simulink model "ClosedLoopControl"  (R2023b)
settings: Solver=FixedStepDiscrete  StartTime=0.0  StopTime=inf  FixedStep=0.005  RelTol=1e-3
libraries: arduinolib x14, arduinosensorlib x4, eeGeneralControl x4, slpidlib x4, embeddedblockslib x2, simulink x2
settings Model: ExtModeTrigDuration=2  Creator=Jakob  LastModifiedBy=Jakob
settings OptimizationCC: EnhancedBackFolding=on  PassReuseOutputArgsAs=Individual arguments  ZeroExternalMemoryAtStartup=off  ZeroInternalMemoryAtStartup=off  MaxStackSize=64  OptimizeBlockOrder=speed  DifferentSizesBufferReuse=on  OptimizationCustomize=off  EfficientTunableParamExpr=on
settings DebuggingCC: ParameterTunabilityLossMsg=error
settings HardwareCC: ProdBitPerPointer=32  ProdBitPerSizeT=32  ProdBitPerPtrDiffT=32  ProdLargestAtomicInteger=Long  ProdLargestAtomicFloat=Double  ProdWordSize=32  ProdHWDeviceType=ARM Compatible->ARM Cortex
settings SFSimCC: MATLABDynamicMemAlloc=off
settings RTWCC: Description=Embedded Coder  SystemTargetFile=ert.tlc  HardwareBoard=ESP32-WROOM(Arduino Compatible)  TLCOptions="-aInlineSetEventsForThisBaseRateFcn=TLC_FALSE -aSuppressMultiTaskScheduler=TLC_FALSE  -aRateBasedStepFcn=0"  TemplateMakefile=ert_default_tmf  Toolchain=ESP32  BuildConfiguration=Faster Runs
settings CodeAppCC: ForceParamTrailComments=on  IgnoreCustomStorageClasses=off  OperatorAnnotations=on  SimulinkDataObjDesc=on  SFDataObjDesc=on  InsertBlockDesc=on
settings ERTTargetCC: SupportContinuousTime=on  SupportVariableSizeSignals=on  ExtModeTransport=3  ExtModeStaticAlloc=on  ExtModeAutomaticAllocSize=off  ExtModeStaticAllocSize=65536  ExtModeMexFile=ext_xcp  ExtModeIntrfLevel=Level2 - Open

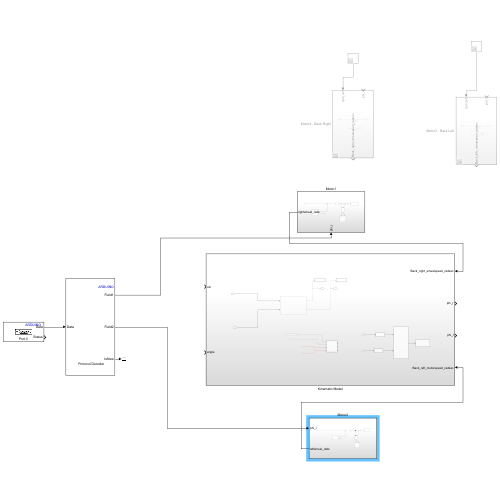
[thumbnail: Simulink's stored preview of the top-level diagram]
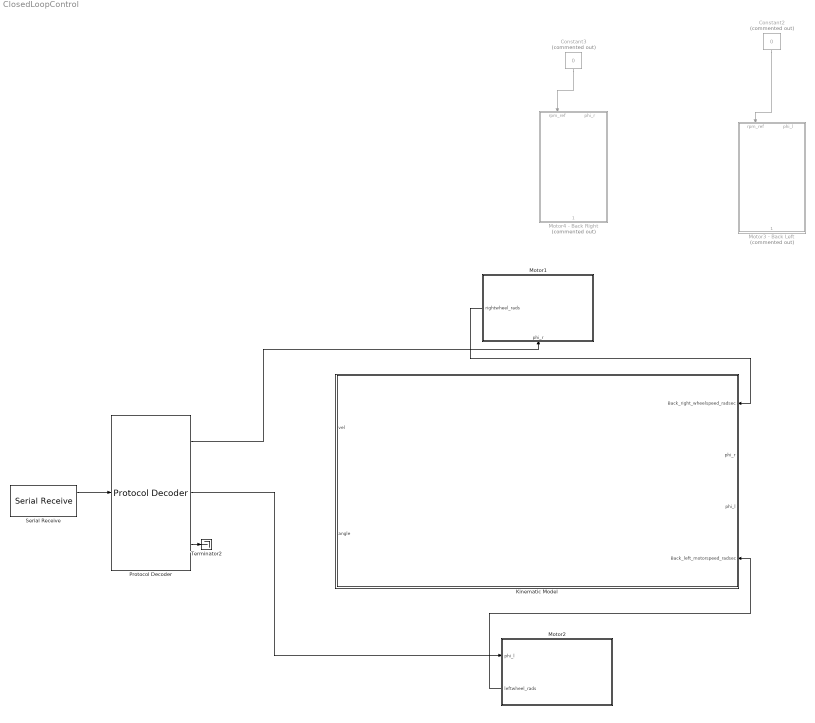
== system ClosedLoopControl ==
  Constant2 : Constant  Commented=on  Value=0
  Constant3 : Constant  Commented=on  Value=0
  Kinematic Model : Subsystem
      settings: PortSchema="{\"entries\":[{\"content\":{\"sides\":[{\"content\":{\"connectorIds\":[\"In1\",\"In2\"]},\"type\":\"ConnectorPlacement.EquallySpacedRectSide\",\"uuid\":\"bea487b3-b9a6-4df2-9051-f476a43b63d0\"},{\"content\":{\"connectorIds\":[\"In3\",\"Out1\",\"Out2\",\"In4\"],\"side\":\"RIGHT\"},\"type\":\"ConnectorPlacement.EquallySpacedRectSide\",\"uuid\":\"7b0ea2f1-f889-4d4a-8825-aa604977931d\"},{\"content\":{\"side\":\"TOP\"},\"type\":\"ConnectorPlacement.EquallySpacedRectSide\",\"uuid\":\"9098ab21-ef51-46af-af75-8fe6529eb13c\"}]},\"type\":\"ConnectorPlacement.EquallySpacedConnector\",\"uuid\":\"e0384f79-f267-486d-9835-e037e5e58d79\"}],\"packageUris\":[\"http://schema.mathworks.com/mf0/Connector/R2020b\"],\"version\":\"1.0\"}"
  Motor1 : Subsystem
      settings: PortSchema="{\"entries\":[{\"content\":{\"sides\":[{\"content\":{},\"type\":\"ConnectorPlacement.EquallySpacedRectSide\",\"uuid\":\"e90522e1-f096-4247-8870-f151728acb54\"},{\"content\":{\"connectorIds\":[\"Out1\"],\"side\":\"RIGHT\"},\"type\":\"ConnectorPlacement.EquallySpacedRectSide\",\"uuid\":\"14a2659e-e07a-4a14-8c7c-2c374d5141ee\"},{\"content\":{\"connectorIds\":[\"In1\"],\"side\":\"TOP\"},\"type\":\"ConnectorPlacement.EquallySpacedRectSide\",\"uuid\":\"95453d09-0c33-4ffa-a097-d1ecacc3e87c\"}]},\"type\":\"ConnectorPlacement.EquallySpacedConnector\",\"uuid\":\"f979addb-97c9-400b-8ed4-2cf1cffe9c36\"}],\"packageUris\":[\"http://schema.mathworks.com/mf0/Connector/R2020b\"],\"version\":\"1.0\"}"
  Motor2 : Subsystem
      settings: PortSchema="{\"entries\":[{\"content\":{\"sides\":[{\"content\":{},\"type\":\"ConnectorPlacement.EquallySpacedRectSide\",\"uuid\":\"e90522e1-f096-4247-8870-f151728acb54\"},{\"content\":{\"connectorIds\":[\"In1\",\"Out1\"],\"side\":\"RIGHT\"},\"type\":\"ConnectorPlacement.EquallySpacedRectSide\",\"uuid\":\"14a2659e-e07a-4a14-8c7c-2c374d5141ee\"},{\"content\":{\"side\":\"TOP\"},\"type\":\"ConnectorPlacement.EquallySpacedRectSide\",\"uuid\":\"95453d09-0c33-4ffa-a097-d1ecacc3e87c\"}]},\"type\":\"ConnectorPlacement.EquallySpacedConnector\",\"uuid\":\"f979addb-97c9-400b-8ed4-2cf1cffe9c36\"}],\"packageUris\":[\"http://schema.mathworks.com/mf0/Connector/R2020b\"],\"version\":\"1.0\"}"
  Motor3 - Back Left : Subsystem  Commented=on
  Motor4 - Back Right : Subsystem  Commented=on
  Protocol Decoder : embeddedblockslib/Protocol Decoder  IsParseCSV=off  Header=['$']  FieldTable={ 'Field1', '1', 'single', 'Little endian'; 'Field2', '1', 'single', 'Little endian' }  IsVariableSizeLastField=off  MaxVariableSizeFieldLength=[]  IsChecksumRequired=off  ChecksumAlgorithm=XOR of bytes  ChecksumSize=[]  TerminatorOption=<none>  CustomTerminatorVal=[]  IsInputLengthAvailable=off  Logo=ARDUINO
      settings: LibrarySourceBlock=arduinolib/Protocol Decoder
  Serial Receive : arduinolib/Serial Receive  isARMArch=off  portNumber=0  DataType=uint8  Datalength=9  SampleTime=0.005  showOutStatus=on  blockPlatform=arduino
  Terminator2 : Terminator
  wires:
  Constant2/1 -> Motor3 - Back Left/1(rpm_ref)
  Constant3/1 -> Motor4 - Back Right/1(rpm_ref)
  Motor2/1(leftwheel_rads) -> Kinematic Model/4(Back_left_motorspeed_radsec)
  Motor1/1(rightwheel_rads) -> Kinematic Model/3(Back_right_wheelspeed_radsec)
  Protocol Decoder/3 -> Terminator2/1
  Serial Receive/1 -> Protocol Decoder/1
  Protocol Decoder/1 -> Motor1/1(phi_r)
  Protocol Decoder/2 -> Motor2/1(phi_l)

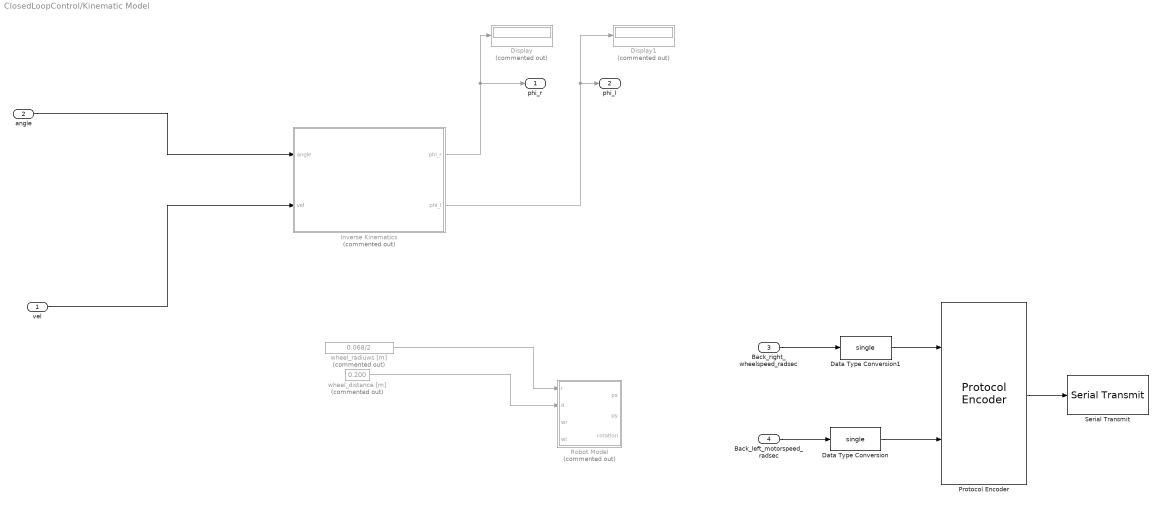
== system ClosedLoopControl/Kinematic Model ==
  vel : Inport
  angle : Inport  Port=2
  Back_right_wheelspeed_radsec : Inport  Port=3
  Back_left_motorspeed_radsec : Inport  Port=4
  Data Type Conversion : DataTypeConversion  OutDataTypeStr=single  SaturateOnIntegerOverflow=off  RndMeth=Floor
  Data Type Conversion1 : DataTypeConversion  OutDataTypeStr=single  SaturateOnIntegerOverflow=off  RndMeth=Floor
  Display : Display  Commented=on
  Display1 : Display  Commented=on
  Inverse Kinematics : Subsystem  Commented=on
  Protocol Encoder : embeddedblockslib/Protocol Encoder  Header=['$']  FieldTable={ 'Field1', '1', 'single', 'Little endian'; 'Field2', '1', 'single', 'Little endian' }  IsChecksumRequired=off  ChecksumAlgorithm=XOR of bytes  ChecksumSize=[]  TerminatorOption=<none>  CustomTerminatorVal=[]  Logo=ARDUINO
      settings: LibrarySourceBlock=arduinolib/Protocol Encoder
  Robot Model : Subsystem  Commented=on
  Serial Transmit : arduinolib/Serial Transmit  portNumber=0  sendmode=write  sendformat=Decimal  floatprecision=2  blockPlatform=arduino
  wheel_distance [m] : Constant  Commented=on  Value=0.200
  wheel_radiuws [m] : Constant  Commented=on  Value=0.068/2
  phi_r : Outport
  phi_l : Outport  Port=2
  wires:
  wheel_radiuws [m]/1 -> Robot Model/1(r)
  wheel_distance [m]/1 -> Robot Model/2(d)
  Inverse Kinematics/1(phi_r) -> Display/1, phi_r/1
  Inverse Kinematics/2(phi_l) -> Display1/1, phi_l/1
  ? -> Robot Model/3(wr)
  ? -> Robot Model/4(wl)
  vel/1 -> Inverse Kinematics/2(vel)
  angle/1 -> Inverse Kinematics/1(angle)
  Protocol Encoder/1 -> Serial Transmit/1
  Data Type Conversion/1 -> Protocol Encoder/2
  Data Type Conversion1/1 -> Protocol Encoder/1
  Back_right_wheelspeed_radsec/1 -> Data Type Conversion1/1
  Back_left_motorspeed_radsec/1 -> Data Type Conversion/1

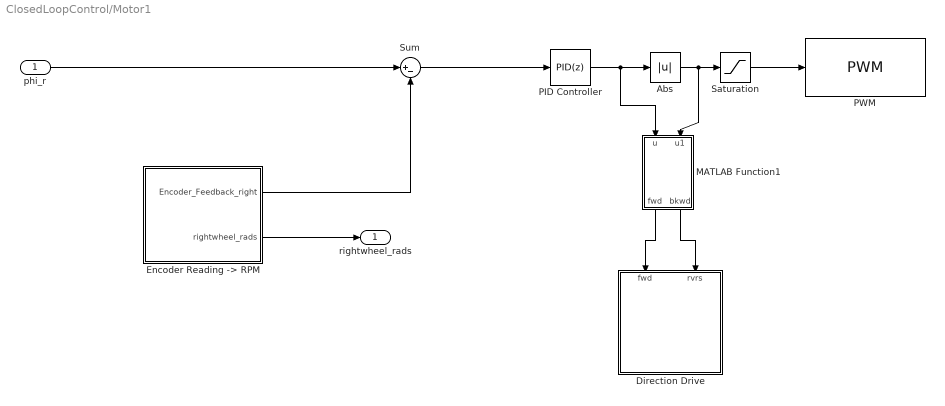
== system ClosedLoopControl/Motor1 ==
  phi_r : Inport
  Abs : Abs  SaturateOnIntegerOverflow=off
  Direction Drive : Subsystem
  "Encoder Reading -> RPM" : Subsystem
  MATLAB Function1 : MATLAB Function  TreatAsAtomicUnit=on
  PID Controller : slpidlib/PID Controller  Controller=PID  Form=Parallel  TimeDomain=Discrete-time  UseExternalTs=off  SampleTime=-1  IntegratorMethod=Forward Euler  FilterMethod=Forward Euler  ControllerParametersSource=internal  P=25  I=350  UseKiTs=off  D=0  N=100  UseFilter=on  TunerSelectOption=Transfer Function Based (PID Tuner App)  InitialConditionSource=internal  InitialConditionForIntegrator=0  InitialConditionForFilter=0  DifferentiatorICPrevScaledInput=0  ExternalReset=none  TrackingMode=off  Kt=1  LimitOutput=off  SatLimitsSource=internal  UpperSaturationLimit=inf  LowerSaturationLimit=-inf  LinearizeAsGain=on  AntiWindupMode=none  Kb=1  LimitIntegrator=off  UpperIntegratorSaturationLimit=inf  LowerIntegratorSaturationLimit=-inf  POutMin=[]  POutMax=[]  IOutMin=[]  IOutMax=[]  DOutMin=[]  DOutMax=[]  NOutMin=[]  NOutMax=[]  SumOutMin=[]  SumOutMax=[]  SaturationOutMin=[]  SaturationOutMax=[]  PParamMin=[]  PParamMax=[]  IParamMin=[]  IParamMax=[]  DParamMin=[]  DParamMax=[]  NParamMin=[]  NParamMax=[]  KbParamMin=[]  KbParamMax=[]  KtParamMin=[]  KtParamMax=[]  KbOutMin=[]  KbOutMax=[]  KtOutMin=[]  KtOutMax=[]  IntegratorOutMin=[]  IntegratorOutMax=[]  FilterOutMin=[]  FilterOutMax=[]  SumI1OutMin=[]  SumI1OutMax=[]  SumI2OutMin=[]  SumI2OutMax=[]  SumI3OutMin=[]  SumI3OutMax=[]  SumI4OutMin=[]  SumI4OutMax=[]  SumDOutMin=[]  SumDOutMax=[]  DifferentiatorOutMin=[]  DifferentiatorOutMax=[]  FilterDiffOutCoefMin=[]  FilterDiffOutCoefMax=[]  ReciprocalOutMin=[]  ReciprocalOutMax=[]  SumDenOutMin=[]  SumDenOutMax=[]  SumNumOutMin=[]  SumNumOutMax=[]  DivideOutMin=[]  DivideOutMax=[]  UdiffTsProdOutMin=[]  UdiffTsProdOutMax=[]  NTsProdOutMin=[]  NTsProdOutMax=[]  UintegralTsProdOutMin=[]  UintegralTsProdOutMax=[]  UngainTsProdOutMin=[]  UngainTsProdOutMax=[]  ClampingZeroOutDataTypeStr=Inherit: Inherit via back propagation  ClampingZeroOutMin=[]  ClampingZeroOutMax=[]  FilterDenConstantOutDataTypeStr=Inherit: Inherit via back propagation  FilterDenConstantOutMin=[]  FilterDenConstantOutMax=[]  PCopyOutDataTypeStr=Inherit: Inherit via back propagation  PCopyOutMin=[]  PCopyOutMax=[]  NCopyOutDataTypeStr=Inherit: Inherit via back propagation  NCopyOutMin=[]  NCopyOutMax=[]  IntegratorContinuousStateAttributes=''  IntegratorStateMustResolveToSignalObject=off  IntegratorRTWStateStorageClass=Auto  FilterContinuousStateAttributes=''  FilterStateMustResolveToSignalObject=off  FilterRTWStateStorageClass=Auto  ParallelPVariant=InternalParameters  IdealPVariant=Disabled  IVariant=InternalParameters  DVariant=InternalParameters  IntegratorVariant=Discrete  SatVariant=Disabled  AWVariant=Passthrough  PCopyVariant=Disabled  TRVariant=Disabled  FdbkBlocksVariant=Forward  IdealPFdbkVariant=Disabled  SatFdbkVariant=Disabled  DerivativeFilterVariant=ForwardEulerFilter  NVariant=InternalParameters  NCopyVariant=Disabled  FilterICVariant=InternalICsFilter  IntegratorICVariant=InternalICs  ExternalResetVariant=Disabled  TRSumVariant=Passthrough  SumFdbkVariant=Disabled  SumVariant=Sum_PID  TsampFilterVariant=InternalTs  TsampNgainVariant=Passthrough  TsampIntegralVariant=Disabled_SignalSpec  ExternalSaturationOutDataTypeStr=Inherit: Same as second input
  PWM : arduinolib/PWM  pinNumber=18  frequencyType=Default  desiredFrequency=490.2  achievableFrequency=490.2
  Saturation : Saturate  UpperLimit=255  LowerLimit=0
  Sum : Sum  Inputs=|+-
  rightwheel_rads : Outport
  wires:
  PID Controller/1 -> MATLAB Function1/1(u), Abs/1
  Sum/1 -> PID Controller/1
  Saturation/1 -> PWM/1
  "Encoder Reading -> RPM"/2(rightwheel_rads) -> rightwheel_rads/1
  phi_r/1 -> Sum/1
  "Encoder Reading -> RPM"/1(Encoder_Feedback_right) -> Sum/2
  Abs/1 -> MATLAB Function1/2(u1), Saturation/1
  MATLAB Function1/1(fwd) -> Direction Drive/1(fwd)
  MATLAB Function1/2(bkwd) -> Direction Drive/2(rvrs)

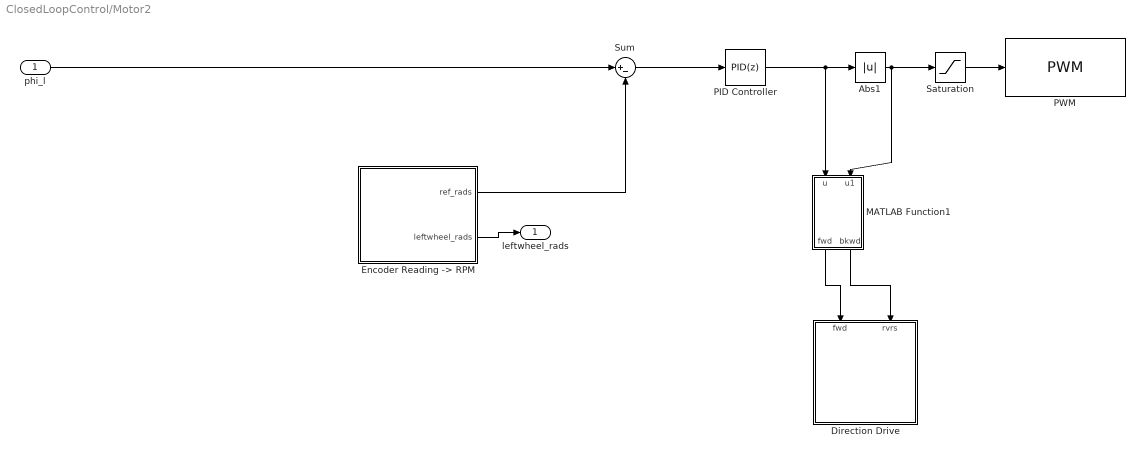
== system ClosedLoopControl/Motor2 ==
  phi_l : Inport
  Abs1 : Abs  SaturateOnIntegerOverflow=off
  Direction Drive : Subsystem
  "Encoder Reading -> RPM" : Subsystem
  MATLAB Function1 : MATLAB Function  TreatAsAtomicUnit=on
  PID Controller : slpidlib/PID Controller  Controller=PID  Form=Parallel  TimeDomain=Discrete-time  UseExternalTs=off  SampleTime=-1  IntegratorMethod=Forward Euler  FilterMethod=Forward Euler  ControllerParametersSource=internal  P=25  I=350  UseKiTs=off  D=0  N=100  UseFilter=on  TunerSelectOption=Transfer Function Based (PID Tuner App)  InitialConditionSource=internal  InitialConditionForIntegrator=0  InitialConditionForFilter=0  DifferentiatorICPrevScaledInput=0  ExternalReset=none  TrackingMode=off  Kt=1  LimitOutput=off  SatLimitsSource=internal  UpperSaturationLimit=inf  LowerSaturationLimit=-inf  LinearizeAsGain=on  AntiWindupMode=none  Kb=1  LimitIntegrator=off  UpperIntegratorSaturationLimit=inf  LowerIntegratorSaturationLimit=-inf  POutMin=[]  POutMax=[]  IOutMin=[]  IOutMax=[]  DOutMin=[]  DOutMax=[]  NOutMin=[]  NOutMax=[]  SumOutMin=[]  SumOutMax=[]  SaturationOutMin=[]  SaturationOutMax=[]  PParamMin=[]  PParamMax=[]  IParamMin=[]  IParamMax=[]  DParamMin=[]  DParamMax=[]  NParamMin=[]  NParamMax=[]  KbParamMin=[]  KbParamMax=[]  KtParamMin=[]  KtParamMax=[]  KbOutMin=[]  KbOutMax=[]  KtOutMin=[]  KtOutMax=[]  IntegratorOutMin=[]  IntegratorOutMax=[]  FilterOutMin=[]  FilterOutMax=[]  SumI1OutMin=[]  SumI1OutMax=[]  SumI2OutMin=[]  SumI2OutMax=[]  SumI3OutMin=[]  SumI3OutMax=[]  SumI4OutMin=[]  SumI4OutMax=[]  SumDOutMin=[]  SumDOutMax=[]  DifferentiatorOutMin=[]  DifferentiatorOutMax=[]  FilterDiffOutCoefMin=[]  FilterDiffOutCoefMax=[]  ReciprocalOutMin=[]  ReciprocalOutMax=[]  SumDenOutMin=[]  SumDenOutMax=[]  SumNumOutMin=[]  SumNumOutMax=[]  DivideOutMin=[]  DivideOutMax=[]  UdiffTsProdOutMin=[]  UdiffTsProdOutMax=[]  NTsProdOutMin=[]  NTsProdOutMax=[]  UintegralTsProdOutMin=[]  UintegralTsProdOutMax=[]  UngainTsProdOutMin=[]  UngainTsProdOutMax=[]  ClampingZeroOutDataTypeStr=Inherit: Inherit via back propagation  ClampingZeroOutMin=[]  ClampingZeroOutMax=[]  FilterDenConstantOutDataTypeStr=Inherit: Inherit via back propagation  FilterDenConstantOutMin=[]  FilterDenConstantOutMax=[]  PCopyOutDataTypeStr=Inherit: Inherit via back propagation  PCopyOutMin=[]  PCopyOutMax=[]  NCopyOutDataTypeStr=Inherit: Inherit via back propagation  NCopyOutMin=[]  NCopyOutMax=[]  IntegratorContinuousStateAttributes=''  IntegratorStateMustResolveToSignalObject=off  IntegratorRTWStateStorageClass=Auto  FilterContinuousStateAttributes=''  FilterStateMustResolveToSignalObject=off  FilterRTWStateStorageClass=Auto  ParallelPVariant=InternalParameters  IdealPVariant=Disabled  IVariant=InternalParameters  DVariant=InternalParameters  IntegratorVariant=Discrete  SatVariant=Disabled  AWVariant=Passthrough  PCopyVariant=Disabled  TRVariant=Disabled  FdbkBlocksVariant=Forward  IdealPFdbkVariant=Disabled  SatFdbkVariant=Disabled  DerivativeFilterVariant=ForwardEulerFilter  NVariant=InternalParameters  NCopyVariant=Disabled  FilterICVariant=InternalICsFilter  IntegratorICVariant=InternalICs  ExternalResetVariant=Disabled  TRSumVariant=Passthrough  SumFdbkVariant=Disabled  SumVariant=Sum_PID  TsampFilterVariant=InternalTs  TsampNgainVariant=Passthrough  TsampIntegralVariant=Disabled_SignalSpec  ExternalSaturationOutDataTypeStr=Inherit: Same as second input
  PWM : arduinolib/PWM  pinNumber=15  frequencyType=Default  desiredFrequency=490.2  achievableFrequency=490.2
  Saturation : Saturate  UpperLimit=255  LowerLimit=0
  Sum : Sum  Inputs=|+-
  leftwheel_rads : Outport
  wires:
  PID Controller/1 -> MATLAB Function1/1(u), Abs1/1
  Sum/1 -> PID Controller/1
  Saturation/1 -> PWM/1
  "Encoder Reading -> RPM"/2(leftwheel_rads) -> leftwheel_rads/1
  phi_l/1 -> Sum/1
  "Encoder Reading -> RPM"/1(ref_rads) -> Sum/2
  Abs1/1 -> MATLAB Function1/2(u1), Saturation/1
  MATLAB Function1/1(fwd) -> Direction Drive/1(fwd)
  MATLAB Function1/2(bkwd) -> Direction Drive/2(rvrs)

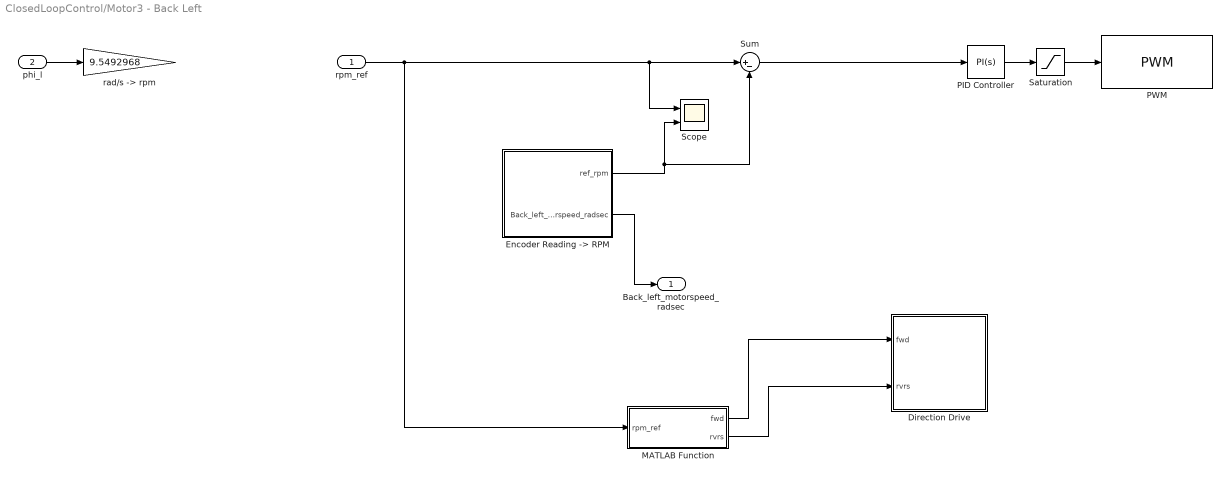
== system ClosedLoopControl/Motor3 - Back Left ==
  rpm_ref : Inport
  phi_l : Inport  Port=2
  Direction Drive : Subsystem
  "Encoder Reading -> RPM" : Subsystem
  MATLAB Function : MATLAB Function  TreatAsAtomicUnit=on
  PID Controller : slpidlib/PID Controller  Controller=PI  Form=Ideal  TimeDomain=Continuous-time  UseExternalTs=off  SampleTime=-1  IntegratorMethod=Forward Euler  FilterMethod=Forward Euler  ControllerParametersSource=internal  P=85  I=0.5  UseKiTs=off  D=0  N=100  UseFilter=on  TunerSelectOption=Transfer Function Based (PID Tuner App)  InitialConditionSource=internal  InitialConditionForIntegrator=0  InitialConditionForFilter=0  DifferentiatorICPrevScaledInput=0  ExternalReset=none  TrackingMode=off  Kt=1  LimitOutput=off  SatLimitsSource=internal  UpperSaturationLimit=inf  LowerSaturationLimit=-inf  LinearizeAsGain=on  AntiWindupMode=none  Kb=1  LimitIntegrator=off  UpperIntegratorSaturationLimit=inf  LowerIntegratorSaturationLimit=-inf  POutMin=[]  POutMax=[]  IOutMin=[]  IOutMax=[]  DOutMin=[]  DOutMax=[]  NOutMin=[]  NOutMax=[]  SumOutMin=[]  SumOutMax=[]  SaturationOutMin=[]  SaturationOutMax=[]  PParamMin=[]  PParamMax=[]  IParamMin=[]  IParamMax=[]  DParamMin=[]  DParamMax=[]  NParamMin=[]  NParamMax=[]  KbParamMin=[]  KbParamMax=[]  KtParamMin=[]  KtParamMax=[]  KbOutMin=[]  KbOutMax=[]  KtOutMin=[]  KtOutMax=[]  IntegratorOutMin=[]  IntegratorOutMax=[]  FilterOutMin=[]  FilterOutMax=[]  SumI1OutMin=[]  SumI1OutMax=[]  SumI2OutMin=[]  SumI2OutMax=[]  SumI3OutMin=[]  SumI3OutMax=[]  SumI4OutMin=[]  SumI4OutMax=[]  SumDOutMin=[]  SumDOutMax=[]  DifferentiatorOutMin=[]  DifferentiatorOutMax=[]  FilterDiffOutCoefMin=[]  FilterDiffOutCoefMax=[]  ReciprocalOutMin=[]  ReciprocalOutMax=[]  SumDenOutMin=[]  SumDenOutMax=[]  SumNumOutMin=[]  SumNumOutMax=[]  DivideOutMin=[]  DivideOutMax=[]  UdiffTsProdOutMin=[]  UdiffTsProdOutMax=[]  NTsProdOutMin=[]  NTsProdOutMax=[]  UintegralTsProdOutMin=[]  UintegralTsProdOutMax=[]  UngainTsProdOutMin=[]  UngainTsProdOutMax=[]  ClampingZeroOutDataTypeStr=Inherit: Inherit via back propagation  ClampingZeroOutMin=[]  ClampingZeroOutMax=[]  FilterDenConstantOutDataTypeStr=Inherit: Inherit via back propagation  FilterDenConstantOutMin=[]  FilterDenConstantOutMax=[]  PCopyOutDataTypeStr=Inherit: Inherit via back propagation  PCopyOutMin=[]  PCopyOutMax=[]  NCopyOutDataTypeStr=Inherit: Inherit via back propagation  NCopyOutMin=[]  NCopyOutMax=[]  IntegratorContinuousStateAttributes=''  IntegratorStateMustResolveToSignalObject=off  IntegratorRTWStateStorageClass=Auto  FilterContinuousStateAttributes=''  FilterStateMustResolveToSignalObject=off  FilterRTWStateStorageClass=Auto  ParallelPVariant=Passthrough  IdealPVariant=InternalParameters  IVariant=InternalParameters  DVariant=Disabled  IntegratorVariant=Continuous  SatVariant=Disabled  AWVariant=Passthrough  PCopyVariant=Disabled  TRVariant=Disabled  FdbkBlocksVariant=Forward  IdealPFdbkVariant=Disabled  SatFdbkVariant=Disabled  DerivativeFilterVariant=Disabled  NVariant=Disabled  NCopyVariant=Disabled_SignalSpec  FilterICVariant=Disabled  IntegratorICVariant=InternalICs  ExternalResetVariant=Disabled  TRSumVariant=Passthrough  SumFdbkVariant=Disabled  SumVariant=Sum_PI  TsampFilterVariant=InternalTs  TsampNgainVariant=Passthrough  TsampIntegralVariant=Disabled_SignalSpec  ExternalSaturationOutDataTypeStr=Inherit: Same as second input
  PWM : arduinolib/PWM  pinNumber=32  frequencyType=Default  desiredFrequency=490.2  achievableFrequency=490.2
  Saturation : Saturate  UpperLimit=255  LowerLimit=-255
  Scope : Scope  NumInputPorts=2
  Sum : Sum  Inputs=|+-
  "rad/s -> rpm" : Gain  Gain=9.5492968
  Back_left_motorspeed_radsec : Outport
  wires:
  PID Controller/1 -> Saturation/1
  Sum/1 -> PID Controller/1
  "Encoder Reading -> RPM"/1(ref_rpm) -> Sum/2, Scope/2
  phi_l/1 -> "rad/s -> rpm"/1
  Saturation/1 -> PWM/1
  "Encoder Reading -> RPM"/2(Back_left_motorspeed_radsec) -> Back_left_motorspeed_radsec/1
  MATLAB Function/1(fwd) -> Direction Drive/1(fwd)
  MATLAB Function/2(rvrs) -> Direction Drive/2(rvrs)
  rpm_ref/1 -> MATLAB Function/1(rpm_ref), Scope/1, Sum/1

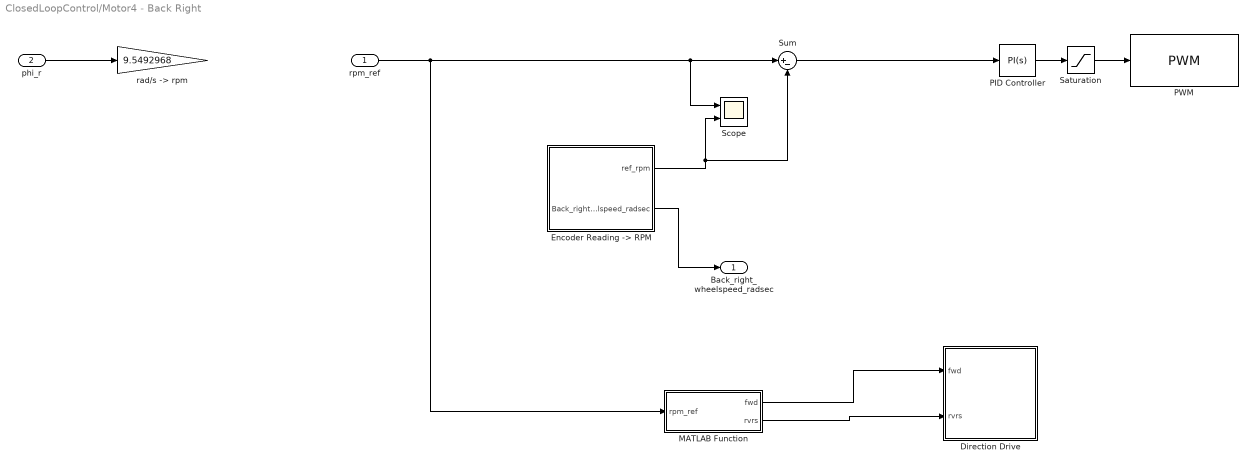
== system ClosedLoopControl/Motor4 - Back Right ==
  rpm_ref : Inport
  phi_r : Inport  Port=2
  Direction Drive : Subsystem
  "Encoder Reading -> RPM" : Subsystem
  MATLAB Function : MATLAB Function  TreatAsAtomicUnit=on
  PID Controller : slpidlib/PID Controller  Controller=PI  Form=Ideal  TimeDomain=Continuous-time  UseExternalTs=off  SampleTime=-1  IntegratorMethod=Forward Euler  FilterMethod=Forward Euler  ControllerParametersSource=internal  P=85  I=0.5  UseKiTs=off  D=0  N=100  UseFilter=on  TunerSelectOption=Transfer Function Based (PID Tuner App)  InitialConditionSource=internal  InitialConditionForIntegrator=0  InitialConditionForFilter=0  DifferentiatorICPrevScaledInput=0  ExternalReset=none  TrackingMode=off  Kt=1  LimitOutput=off  SatLimitsSource=internal  UpperSaturationLimit=inf  LowerSaturationLimit=-inf  LinearizeAsGain=on  AntiWindupMode=none  Kb=1  LimitIntegrator=off  UpperIntegratorSaturationLimit=inf  LowerIntegratorSaturationLimit=-inf  POutMin=[]  POutMax=[]  IOutMin=[]  IOutMax=[]  DOutMin=[]  DOutMax=[]  NOutMin=[]  NOutMax=[]  SumOutMin=[]  SumOutMax=[]  SaturationOutMin=[]  SaturationOutMax=[]  PParamMin=[]  PParamMax=[]  IParamMin=[]  IParamMax=[]  DParamMin=[]  DParamMax=[]  NParamMin=[]  NParamMax=[]  KbParamMin=[]  KbParamMax=[]  KtParamMin=[]  KtParamMax=[]  KbOutMin=[]  KbOutMax=[]  KtOutMin=[]  KtOutMax=[]  IntegratorOutMin=[]  IntegratorOutMax=[]  FilterOutMin=[]  FilterOutMax=[]  SumI1OutMin=[]  SumI1OutMax=[]  SumI2OutMin=[]  SumI2OutMax=[]  SumI3OutMin=[]  SumI3OutMax=[]  SumI4OutMin=[]  SumI4OutMax=[]  SumDOutMin=[]  SumDOutMax=[]  DifferentiatorOutMin=[]  DifferentiatorOutMax=[]  FilterDiffOutCoefMin=[]  FilterDiffOutCoefMax=[]  ReciprocalOutMin=[]  ReciprocalOutMax=[]  SumDenOutMin=[]  SumDenOutMax=[]  SumNumOutMin=[]  SumNumOutMax=[]  DivideOutMin=[]  DivideOutMax=[]  UdiffTsProdOutMin=[]  UdiffTsProdOutMax=[]  NTsProdOutMin=[]  NTsProdOutMax=[]  UintegralTsProdOutMin=[]  UintegralTsProdOutMax=[]  UngainTsProdOutMin=[]  UngainTsProdOutMax=[]  ClampingZeroOutDataTypeStr=Inherit: Inherit via back propagation  ClampingZeroOutMin=[]  ClampingZeroOutMax=[]  FilterDenConstantOutDataTypeStr=Inherit: Inherit via back propagation  FilterDenConstantOutMin=[]  FilterDenConstantOutMax=[]  PCopyOutDataTypeStr=Inherit: Inherit via back propagation  PCopyOutMin=[]  PCopyOutMax=[]  NCopyOutDataTypeStr=Inherit: Inherit via back propagation  NCopyOutMin=[]  NCopyOutMax=[]  IntegratorContinuousStateAttributes=''  IntegratorStateMustResolveToSignalObject=off  IntegratorRTWStateStorageClass=Auto  FilterContinuousStateAttributes=''  FilterStateMustResolveToSignalObject=off  FilterRTWStateStorageClass=Auto  ParallelPVariant=Passthrough  IdealPVariant=InternalParameters  IVariant=InternalParameters  DVariant=Disabled  IntegratorVariant=Continuous  SatVariant=Disabled  AWVariant=Passthrough  PCopyVariant=Disabled  TRVariant=Disabled  FdbkBlocksVariant=Forward  IdealPFdbkVariant=Disabled  SatFdbkVariant=Disabled  DerivativeFilterVariant=Disabled  NVariant=Disabled  NCopyVariant=Disabled_SignalSpec  FilterICVariant=Disabled  IntegratorICVariant=InternalICs  ExternalResetVariant=Disabled  TRSumVariant=Passthrough  SumFdbkVariant=Disabled  SumVariant=Sum_PI  TsampFilterVariant=InternalTs  TsampNgainVariant=Passthrough  TsampIntegralVariant=Disabled_SignalSpec  ExternalSaturationOutDataTypeStr=Inherit: Same as second input
  PWM : arduinolib/PWM  pinNumber=13  frequencyType=Default  desiredFrequency=490.2  achievableFrequency=490.2
  Saturation : Saturate  UpperLimit=255  LowerLimit=-255
  Scope : Scope  NumInputPorts=2
  Sum : Sum  Inputs=|+-
  "rad/s -> rpm" : Gain  Gain=9.5492968
  Back_right_wheelspeed_radsec : Outport
  wires:
  PID Controller/1 -> Saturation/1
  Sum/1 -> PID Controller/1
  "Encoder Reading -> RPM"/1(ref_rpm) -> Sum/2, Scope/2
  phi_r/1 -> "rad/s -> rpm"/1
  Saturation/1 -> PWM/1
  "Encoder Reading -> RPM"/2(Back_right_wheelspeed_radsec) -> Back_right_wheelspeed_radsec/1
  MATLAB Function/1(fwd) -> Direction Drive/1(fwd)
  MATLAB Function/2(rvrs) -> Direction Drive/2(rvrs)
  rpm_ref/1 -> MATLAB Function/1(rpm_ref), Scope/1, Sum/1

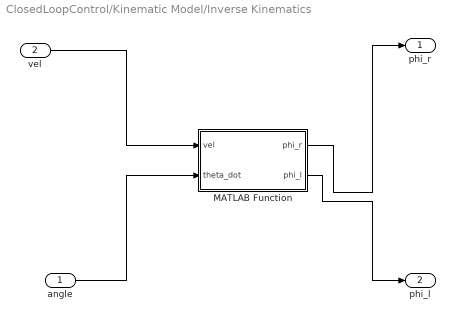
== system ClosedLoopControl/Kinematic Model/Inverse Kinematics ==
  angle : Inport
  vel : Inport  Port=2
  MATLAB Function : MATLAB Function  TreatAsAtomicUnit=on
  phi_r : Outport
  phi_l : Outport  Port=2
  wires:
  angle/1 -> MATLAB Function/2(theta_dot)
  vel/1 -> MATLAB Function/1(vel)
  MATLAB Function/1(phi_r) -> phi_r/1
  MATLAB Function/2(phi_l) -> phi_l/1

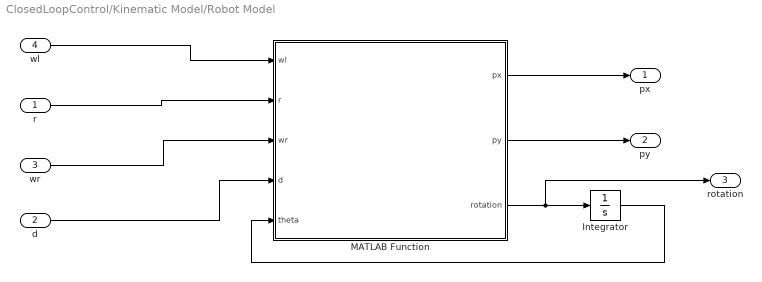
== system ClosedLoopControl/Kinematic Model/Robot Model ==
  r : Inport
  d : Inport  Port=2
  wr : Inport  Port=3
  wl : Inport  Port=4
  Integrator : Integrator
  MATLAB Function : MATLAB Function  TreatAsAtomicUnit=on
  px : Outport
  py : Outport  Port=2
  rotation : Outport  Port=3
  wires:
  wl/1 -> MATLAB Function/1(wl)
  r/1 -> MATLAB Function/2(r)
  d/1 -> MATLAB Function/4(d)
  wr/1 -> MATLAB Function/3(wr)
  MATLAB Function/1(px) -> px/1
  MATLAB Function/2(py) -> py/1
  MATLAB Function/3(rotation) -> rotation/1, Integrator/1
  Integrator/1 -> MATLAB Function/5(theta)

== system ClosedLoopControl/Motor1/Direction Drive ==
  fwd : Inport
  rvrs : Inport  Port=2
  Forward : arduinolib/Digital Output  pinNumber=5  Direction=output  blockPlatform=arduino
  Reverse : arduinolib/Digital Output  pinNumber=17  Direction=output  blockPlatform=arduino
  wires:
  rvrs/1 -> Reverse/1
  fwd/1 -> Forward/1

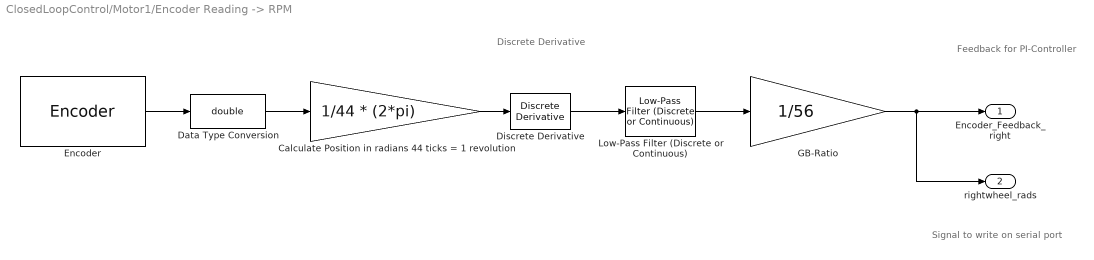
== system ClosedLoopControl/Motor1/Encoder Reading -> RPM ==
  note: Signal to write on serial port
  note: Feedback for PI-Controller
  note: Discrete Derivative
  Calculate Position in radians 44 ticks = 1 revolution : Gain  Gain=1/44 * (2*pi)
  Data Type Conversion : DataTypeConversion  OutDataTypeStr=double  SaturateOnIntegerOverflow=off  RndMeth=Floor
  Discrete Derivative : simulink/Discrete/Discrete Derivative  gainval=1.0  ICPrevScaledInput=0.0  OutMin=[]  OutMax=[]  OutDataType=fixdt(1, 16)  OutScaling=2^-10  DoSatur=off
  Encoder : arduinosensorlib/Encoder  InputA=19  InputB=23  Mode=No reset  SampleTime=-1
  GB-Ratio : Gain  Gain=1/56
  Low-Pass Filter (Discrete or Continuous) : eeGeneralControl/Low-Pass Filter (Discrete or Continuous)  K=1  T=0.05  B=inf  A=-inf  init_option=Inherited from block input  x0=0  Ts=-1
  Encoder_Feedback_right : Outport
  rightwheel_rads : Outport  Port=2
  wires:
  Calculate Position in radians 44 ticks = 1 revolution/1 -> Discrete Derivative/1
  Encoder/1 -> Data Type Conversion/1
  Data Type Conversion/1 -> Calculate Position in radians 44 ticks = 1 revolution/1
  Discrete Derivative/1 -> Low-Pass Filter (Discrete or Continuous)/1
  GB-Ratio/1 -> Encoder_Feedback_right/1, rightwheel_rads/1
  Low-Pass Filter (Discrete or Continuous)/1 -> GB-Ratio/1

== system ClosedLoopControl/Motor2/Direction Drive ==
  fwd : Inport
  rvrs : Inport  Port=2
  Forward : arduinolib/Digital Output  pinNumber=22  Direction=output  blockPlatform=arduino
  Reverse : arduinolib/Digital Output  pinNumber=2  Direction=output  blockPlatform=arduino
  wires:
  rvrs/1 -> Reverse/1
  fwd/1 -> Forward/1

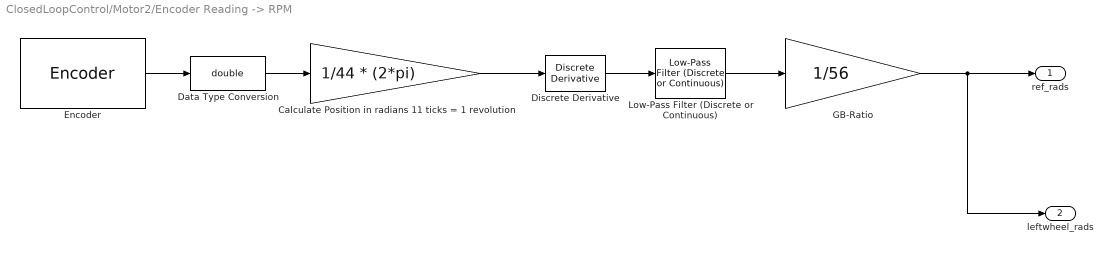
== system ClosedLoopControl/Motor2/Encoder Reading -> RPM ==
  Calculate Position in radians 11 ticks = 1 revolution : Gain  Gain=1/44 * (2*pi)
  Data Type Conversion : DataTypeConversion  OutDataTypeStr=double  SaturateOnIntegerOverflow=off  RndMeth=Floor
  Discrete Derivative : simulink/Discrete/Discrete Derivative  gainval=1.0  ICPrevScaledInput=0.0  OutMin=[]  OutMax=[]  OutDataType=fixdt(1, 16)  OutScaling=2^-10  DoSatur=off
  Encoder : arduinosensorlib/Encoder  InputA=4  InputB=16  Mode=No reset  SampleTime=-1
  GB-Ratio : Gain  Gain=1/56
  Low-Pass Filter (Discrete or Continuous) : eeGeneralControl/Low-Pass Filter (Discrete or Continuous)  K=1  T=0.05  B=inf  A=-inf  init_option=Inherited from block input  x0=0  Ts=-1
  ref_rads : Outport
  leftwheel_rads : Outport  Port=2
  wires:
  Calculate Position in radians 11 ticks = 1 revolution/1 -> Discrete Derivative/1
  Encoder/1 -> Data Type Conversion/1
  Data Type Conversion/1 -> Calculate Position in radians 11 ticks = 1 revolution/1
  Discrete Derivative/1 -> Low-Pass Filter (Discrete or Continuous)/1
  GB-Ratio/1 -> ref_rads/1, leftwheel_rads/1
  Low-Pass Filter (Discrete or Continuous)/1 -> GB-Ratio/1

== system ClosedLoopControl/Motor3 - Back Left/Direction Drive ==
  fwd : Inport
  rvrs : Inport  Port=2
  Forward : arduinolib/Digital Output  pinNumber=25  Direction=output  blockPlatform=arduino
  Reverse : arduinolib/Digital Output  pinNumber=33  Direction=output  blockPlatform=arduino
  wires:
  rvrs/1 -> Reverse/1
  fwd/1 -> Forward/1

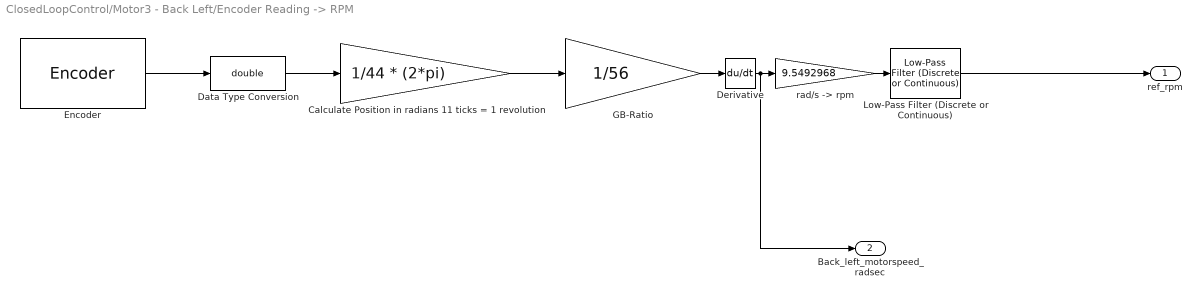
== system ClosedLoopControl/Motor3 - Back Left/Encoder Reading -> RPM ==
  Calculate Position in radians 11 ticks = 1 revolution : Gain  Gain=1/44 * (2*pi)
  Data Type Conversion : DataTypeConversion  OutDataTypeStr=double  SaturateOnIntegerOverflow=off  RndMeth=Floor
  Derivative : Derivative
  Encoder : arduinosensorlib/Encoder  InputA=34  InputB=35  Mode=No reset  SampleTime=-1
  GB-Ratio : Gain  Gain=1/56
  Low-Pass Filter (Discrete or Continuous) : eeGeneralControl/Low-Pass Filter (Discrete or Continuous)  K=1  T=0.5  B=inf  A=-inf  init_option=Inherited from block input  x0=0  Ts=-1
  "rad/s -> rpm" : Gain  Gain=9.5492968
  ref_rpm : Outport
  Back_left_motorspeed_radsec : Outport  Port=2
  wires:
  Calculate Position in radians 11 ticks = 1 revolution/1 -> GB-Ratio/1
  Encoder/1 -> Data Type Conversion/1
  Data Type Conversion/1 -> Calculate Position in radians 11 ticks = 1 revolution/1
  GB-Ratio/1 -> Derivative/1
  Derivative/1 -> Back_left_motorspeed_radsec/1, "rad/s -> rpm"/1
  "rad/s -> rpm"/1 -> Low-Pass Filter (Discrete or Continuous)/1
  Low-Pass Filter (Discrete or Continuous)/1 -> ref_rpm/1

== system ClosedLoopControl/Motor4 - Back Right/Direction Drive ==
  fwd : Inport
  rvrs : Inport  Port=2
  Forward : arduinolib/Digital Output  pinNumber=12  Direction=output  blockPlatform=arduino
  Reverse : arduinolib/Digital Output  pinNumber=14  Direction=output  blockPlatform=arduino
  wires:
  rvrs/1 -> Reverse/1
  fwd/1 -> Forward/1

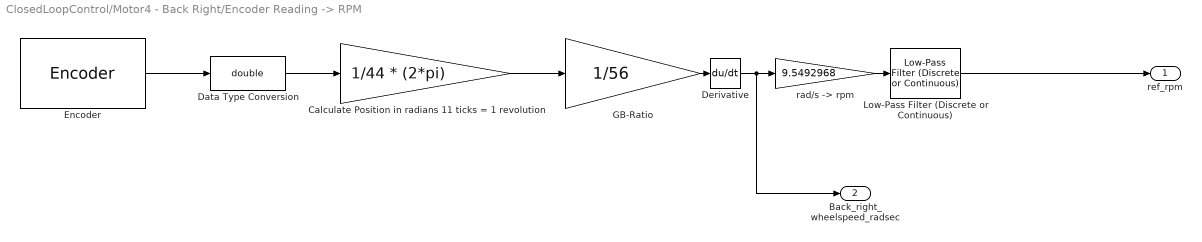
== system ClosedLoopControl/Motor4 - Back Right/Encoder Reading -> RPM ==
  Calculate Position in radians 11 ticks = 1 revolution : Gain  Gain=1/44 * (2*pi)
  Data Type Conversion : DataTypeConversion  OutDataTypeStr=double  SaturateOnIntegerOverflow=off  RndMeth=Floor
  Derivative : Derivative
  Encoder : arduinosensorlib/Encoder  InputA=26  InputB=27  Mode=No reset  SampleTime=-1
  GB-Ratio : Gain  Gain=1/56
  Low-Pass Filter (Discrete or Continuous) : eeGeneralControl/Low-Pass Filter (Discrete or Continuous)  K=1  T=0.5  B=inf  A=-inf  init_option=Inherited from block input  x0=0  Ts=-1
  "rad/s -> rpm" : Gain  Gain=9.5492968
  ref_rpm : Outport
  Back_right_wheelspeed_radsec : Outport  Port=2
  wires:
  Calculate Position in radians 11 ticks = 1 revolution/1 -> GB-Ratio/1
  Encoder/1 -> Data Type Conversion/1
  Data Type Conversion/1 -> Calculate Position in radians 11 ticks = 1 revolution/1
  GB-Ratio/1 -> Derivative/1
  Derivative/1 -> Back_right_wheelspeed_radsec/1, "rad/s -> rpm"/1
  "rad/s -> rpm"/1 -> Low-Pass Filter (Discrete or Continuous)/1
  Low-Pass Filter (Discrete or Continuous)/1 -> ref_rpm/1

== matlab function ClosedLoopControl/Kinematic Model/Robot Model/MATLAB Function ==
  data: wl input; px output; r input; wr input; d input; py output; rotation output; theta input
function [px,py,rotation] = fcn(wl,r,wr,d,theta)

mat1 = [r/2, r/2;0,0;r/(2*d),-r/(2*d)];
mat2 = [wr;wl];

T1=[cos(theta), sin(theta),0;-sin(theta),cos(theta),0;0,0,1];
m = mat1*mat2;

m_m= T1*m;
px = m_m(1,1);
py = m_m(2,1);
rotation  = m_m(3,1);

== matlab function ClosedLoopControl/Kinematic Model/Inverse Kinematics/MATLAB Function ==
  data: vel input; phi_r output; theta_dot input; phi_l output
function [phi_r, phi_l]= fcn(vel, theta_dot)

r= 0.068/2; % Must be changed to fit UiABot
d= 0.200;

%T1=[cos(theta), -sin(theta),0;sin(theta),cos(theta),0;0,0,1];

mat1 = [1/r,0,d/r; 1/r,0,-d/r];

mat2=[vel;0;theta_dot];

M = mat1*mat2; 

%m_m = T1*M;

phi_r=M(1,1);
phi_l=M(2,1);

== matlab function ClosedLoopControl/Motor4 - Back Right/MATLAB Function ==
  data: rpm_ref input; fwd output; rvrs output
function [fwd, rvrs] = fcn(rpm_ref)

fwd = 0;
rvrs = 0;
if rpm_ref > 0
    fwd = 1;
    rvrs = 0;
elseif rpm_ref < 0
    fwd = 0;
    rvrs = 1;
else
    fwd = 0;
    rvrs = 0;
end

== matlab function ClosedLoopControl/Motor3 - Back Left/MATLAB Function ==
  data: rpm_ref input; fwd output; rvrs output
function [fwd, rvrs] = fcn(rpm_ref)

fwd = 0;
rvrs = 0;
if rpm_ref > 0
    fwd = 1;
    rvrs = 0;
elseif rpm_ref < 0
    fwd = 0;
    rvrs = 1;
else
    fwd = 0;
    rvrs = 0;
end

== matlab function ClosedLoopControl/Motor2/MATLAB Function1 ==
  data: u input; fwd output; bkwd output; u1 input
function [fwd, bkwd] = fcn(u, u1)

if(u > 0)
    fwd = 1;
    bkwd = 0;
    if(u1 < 90)
        fwd = 0;
        bkwd = 0;
    end
else
    fwd = 0;
    bkwd = 1;
    if(u1 < 90)
        fwd = 0;
        bkwd = 0;
    end
end

== matlab function ClosedLoopControl/Motor1/MATLAB Function1 ==
  data: u input; fwd output; bkwd output; u1 input
function [fwd, bkwd] = fcn(u, u1)

if(u > 0)
    fwd = 1;
    bkwd = 0;
    if(u1 < 90)
        fwd = 0;
        bkwd = 0;
    end
else
    fwd = 0;
    bkwd = 1;
    if(u1 < 90)
        fwd = 0;
        bkwd = 0;
    end
end
